simulink library "mag_logic_lib"  (R2016b)
settings: Solver=VariableStepAuto  StartTime=0.0  StopTime=10.0  RelTol=1e-3
undefined symbols (not defined in the file or in its folder): fsw_params
libraries: single_2_bool x1
settings Model: Creator=Taylor  LastModifiedBy=Taylor

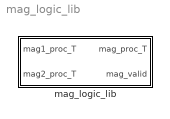
== system mag_logic_lib ==
  mag_logic_lib : Subsystem

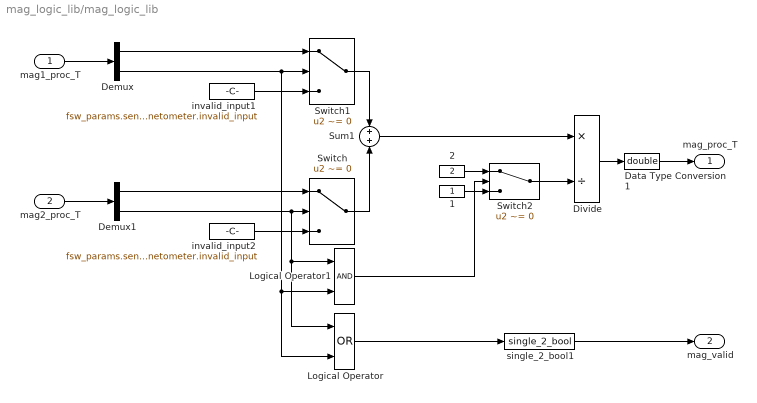
== system mag_logic_lib/mag_logic_lib ==
  mag1_proc_T : Inport
  mag2_proc_T : Inport  Port=2
  1 : Constant  OutDataTypeStr=single  SampleTime=fsw_params.sample_time_s
  2 : Constant  Value=2  OutDataTypeStr=single  SampleTime=fsw_params.sample_time_s
  Data Type Conversion1 : DataTypeConversion  OutDataTypeStr=double
  Demux : Demux  Outputs=[3 1]
  Demux1 : Demux  Outputs=[3 1]
  Divide : Product  Inputs=*/
  Logical Operator : Logic  Operator=OR  AllPortsSameDT=off  OutDataTypeStr=boolean
  Logical Operator1 : Logic  AllPortsSameDT=off  OutDataTypeStr=boolean
  Sum1 : Sum
  Switch : Switch  Criteria=u2 ~= 0
  Switch1 : Switch  Criteria=u2 ~= 0
  Switch2 : Switch  Criteria=u2 ~= 0
  "invalid_input1 " : Constant  Value=fsw_params.sensor_processing.magnetometer.invalid_input  OutDataTypeStr=single  SampleTime=fsw_params.sample_time_s
  invalid_input2 : Constant  Value=fsw_params.sensor_processing.magnetometer.invalid_input  OutDataTypeStr=single  SampleTime=fsw_params.sample_time_s
  single_2_bool1 : single_2_bool/single_2_bool
  mag_proc_T : Outport
  mag_valid : Outport  Port=2
  wires:
  Switch2/1 -> Divide/2
  1/1 -> Switch2/3
  2/1 -> Switch2/1
  Logical Operator1/1 -> Switch2/2
  Sum1/1 -> Divide/1
  Switch1/1 -> Sum1/1
  Switch/1 -> Sum1/2
  "invalid_input1 "/1 -> Switch1/3
  Demux/1 -> Switch1/1
  invalid_input2/1 -> Switch/3
  Demux1/1 -> Switch/1
  Demux1/2 -> Switch/2, Logical Operator1/1, Logical Operator/1
  Demux/2 -> Logical Operator1/2, Logical Operator/2, Switch1/2
  Divide/1 -> Data Type Conversion1/1
  mag1_proc_T/1 -> Demux/1
  mag2_proc_T/1 -> Demux1/1
  Logical Operator/1 -> single_2_bool1/1
  Data Type Conversion1/1 -> mag_proc_T/1
  single_2_bool1/1 -> mag_valid/1
